simulink model "PR_Planar_Testbench_2018"  (R2024a)
settings: Solver=FixedStepDiscrete  StartTime=0.0  StopTime=inf  FixedStep=param.t_sample  RelTol=1e-3
undefined symbols (not defined in the file): max_qa, min_qa, param, slave3
libraries: Cust_Library_planarPKM x54, simulink_extras x27, dspswit3 x24, simulink x22, etherlab_lib x12
(part 5 of 6)

== system PR_Planar_Testbench_2018/Communication/Klemmen zu Simulink/int in double1 ==
  pos_raw : Inport
  current_raw : Inport  Port=2
  Constant : Constant  Value=param.t_sample  SampleTime=-1
  Delay1 : Delay  DelayLength=1  InitialCondition=param.offset_qa2_rad
  Delay4 : Delay  DelayLength=1
  MATLAB Function1 : MATLAB Function  TreatAsAtomicUnit=on
  Position_i1 : Gain  Gain=(2*pi)/(2^(20))  ParamDataTypeStr=float('double')  OutDataTypeStr=float('double')
  Sum1 : Sum  Inputs=|+-
  Torque_i1 : Gain  Gain=(6.6116*16.5)/3280  ParamDataTypeStr=float('double')  OutDataTypeStr=float('double')
  int16_2_double : DataTypeConversion  OutDataTypeStr=double  SaturateOnIntegerOverflow=off  RndMeth=Floor
  offset_s1 : Constant  Value=param.offset_qa2_rad  SampleTime=-1
  pos_Achse12 : DataTypeConversion  OutDataTypeStr=double  SaturateOnIntegerOverflow=off  RndMeth=Floor
  pos : Outport
  vel : Outport  Port=2
  acc : Outport  Port=3
  tau : Outport  Port=4
  wires:
  current_raw/1 -> int16_2_double/1
  Constant/1 -> MATLAB Function1/4(t_sample)
  Delay4/1 -> MATLAB Function1/3(prev_vel)
  pos_raw/1 -> pos_Achse12/1
  MATLAB Function1/1(vel) -> Delay4/1, vel/1  "dq"
  Delay1/1 -> MATLAB Function1/2(prev_pos)
  MATLAB Function1/2(acc) -> acc/1
  Torque_i1/1 -> tau/1  "tau_mess_RD1"
  pos_Achse12/1 -> Position_i1/1
  offset_s1/1 -> Sum1/2
  Position_i1/1 -> Sum1/1
  Sum1/1 -> pos/1, Delay1/1, MATLAB Function1/1(u)
  int16_2_double/1 -> Torque_i1/1

== system PR_Planar_Testbench_2018/Communication/Klemmen zu Simulink/int in double2 ==
  pos_raw : Inport
  current_raw : Inport  Port=2
  Constant : Constant  Value=param.t_sample  SampleTime=-1
  Delay1 : Delay  DelayLength=1  InitialCondition=param.offset_qa3_rad
  Delay4 : Delay  DelayLength=1
  MATLAB Function1 : MATLAB Function  TreatAsAtomicUnit=on
  Position_i1 : Gain  Gain=(2*pi)/(2^(20))  ParamDataTypeStr=float('double')  OutDataTypeStr=float('double')
  Sum1 : Sum  Inputs=|+-
  Torque_i1 : Gain  Gain=(6.7315*16.5)/3280  ParamDataTypeStr=float('double')  OutDataTypeStr=float('double')
  int16_2_double : DataTypeConversion  OutDataTypeStr=double  SaturateOnIntegerOverflow=off  RndMeth=Floor
  offset_s1 : Constant  Value=param.offset_qa3_rad  SampleTime=-1
  pos_Achse12 : DataTypeConversion  OutDataTypeStr=double  SaturateOnIntegerOverflow=off  RndMeth=Floor
  pos : Outport
  vel : Outport  Port=2
  acc : Outport  Port=3
  tau : Outport  Port=4
  wires:
  current_raw/1 -> int16_2_double/1
  Constant/1 -> MATLAB Function1/4(t_sample)
  Delay4/1 -> MATLAB Function1/3(prev_vel)
  pos_raw/1 -> pos_Achse12/1
  MATLAB Function1/1(vel) -> Delay4/1, vel/1  "dq"
  Delay1/1 -> MATLAB Function1/2(prev_pos)
  MATLAB Function1/2(acc) -> acc/1
  Torque_i1/1 -> tau/1  "tau_mess_RD1"
  pos_Achse12/1 -> Position_i1/1
  offset_s1/1 -> Sum1/2
  Position_i1/1 -> Sum1/1
  Sum1/1 -> pos/1, Delay1/1, MATLAB Function1/1(u)
  int16_2_double/1 -> Torque_i1/1

== system PR_Planar_Testbench_2018/Logic/Trajectory/Acceleration ==
  tr_run : Inport
  Counter : Inport  Port=2
  traj_length : Inport  Port=3
  Constant1 : Constant  Value=0  SampleTime=-1
  Less Than : RelationalOperator  Operator=<  OutDataTypeStr=boolean  RndMeth=Simplest  InputSameDT=off
  Mux : Mux  Inputs=3
  OR : Logic  AllPortsSameDT=off  OutDataTypeStr=boolean
  PhieDD : Constant  Value=0  SampleTime=-1
  Saturation : Saturate  UpperLimit=param.len_traj_init-1  LowerLimit=0
  Selector : Selector  IndexMode=Zero-based  IndexOptions=Index vector (port)  Indices=[1 3]  OutputSizes=1
  Selector1 : Selector  IndexMode=Zero-based  IndexOptions=Index vector (port)  Indices=[1 3]  OutputSizes=1
  Selector2 : Selector  IndexMode=Zero-based  IndexOptions=Index vector (port)  Indices=[1 3]  OutputSizes=1
  Switch : Switch  Criteria=u2 > Threshold  SaturateOnIntegerOverflow=off  InputSameDT=off
  XDD : Constant  Value=0  SampleTime=-1
  YDD : Constant  Value=0  SampleTime=-1
  XDDE_soll : Outport
  wires:
  Constant1/1 -> Switch/3
  traj_length/1 -> Less Than/2
  Selector2/1 -> Mux/3
  PhieDD/1 -> Selector2/1
  Selector1/1 -> Mux/2
  Counter/1 -> Switch/1, Less Than/1
  XDD/1 -> Selector/1
  Switch/1 -> Saturation/1
  Less Than/1 -> OR/2
  OR/1 -> Switch/2
  Selector/1 -> Mux/1
  YDD/1 -> Selector1/1
  Mux/1 -> XDDE_soll/1
  tr_run/1 -> OR/1
  Saturation/1 -> Selector2/2, Selector1/2, Selector/2

== system PR_Planar_Testbench_2018/Logic/Trajectory/Pose ==
  tr_run : Inport
  Counter : Inport  Port=2
  traj_length : Inport  Port=3
  AND : Logic  AllPortsSameDT=off  OutDataTypeStr=boolean
  AND1 : Logic  AllPortsSameDT=off  OutDataTypeStr=boolean
  Constant1 : Constant  Value=0  SampleTime=-1
  Constant5 : Constant  Value=0  SampleTime=-1
  Delay1 : Delay  DelayLength=1
  Equal : RelationalOperator  Operator=~=  OutDataTypeStr=boolean  RndMeth=Simplest  InputSameDT=off
  Less Than : RelationalOperator  Operator=<  OutDataTypeStr=boolean  RndMeth=Simplest  InputSameDT=off
  Mux : Mux  Inputs=3
  Mux1 : Mux  Inputs=3
  Phie : Constant  Value=0  SampleTime=-1
  Phie0 : Constant  Value=0  SampleTime=-1
  Saturation : Saturate  UpperLimit=param.len_traj_init-1  LowerLimit=0
  Scope : Scope  NumInputPorts=2
  Scope1 : Scope  NumInputPorts=3
  Scope2 : Scope  NumInputPorts=2
  Scope3 : Scope
  Selector{,1..3} (4 alike) : Selector  IndexMode=Zero-based  IndexOptions=Index vector (port)  Indices=[1 3]  OutputSizes=1
  Switch : Switch  Criteria=u2 > Threshold  SaturateOnIntegerOverflow=off  InputSameDT=off
  X : Constant  Value=0  SampleTime=-1
  X0 : Constant  Value=0  SampleTime=-1
  Y : Constant  Value=0  SampleTime=-1
  Y0 : Constant  Value=0  SampleTime=-1
  isValid : Constant  Value=0  SampleTime=-1
  XE_soll : Outport
  tr_isCalculating : Outport  Port=2
  XE0_soll : Outport  Port=3
  tr_valid : Outport  Port=4
  wires:
  Constant1/1 -> Switch/3
  traj_length/1 -> Less Than/2
  Selector2/1 -> Mux/3
  Phie/1 -> Selector2/1
  Selector1/1 -> Mux/2
  Counter/1 -> Scope1/1, Switch/1, Less Than/1, Scope3/1
  Selector/1 -> Mux/1
  Constant5/1 -> Equal/1
  Switch/1 -> Saturation/1, Equal/2
  Less Than/1 -> Scope1/3, AND/2
  AND/1 -> Switch/2
  Mux/1 -> XE_soll/1
  Mux1/1 -> XE0_soll/1
  Equal/1 -> Scope2/2, AND1/2
  Y/1 -> Selector1/1
  tr_run/1 -> Scope1/2, AND/1, Scope2/1, AND1/1
  Y0/1 -> Mux1/2
  X0/1 -> Mux1/1
  Phie0/1 -> Mux1/3
  Saturation/1 -> Scope/2, Selector3/2, Selector/2, Selector1/2, Selector2/2
  AND1/1 -> tr_isCalculating/1, Scope/1
  X/1 -> Selector/1
  isValid/1 -> Selector3/1
  Selector3/1 -> Delay1/1
  Delay1/1 -> tr_valid/1

== system PR_Planar_Testbench_2018/Logic/Trajectory/Velocity ==
  tr_run : Inport
  Counter : Inport  Port=2
  traj_length : Inport  Port=3
  Constant1 : Constant  Value=0  SampleTime=-1
  Display : Display
  Less Than : RelationalOperator  Operator=<  OutDataTypeStr=boolean  RndMeth=Simplest  InputSameDT=off
  Mux : Mux  Inputs=3
  OR : Logic  AllPortsSameDT=off  OutDataTypeStr=boolean
  PhieD : Constant  Value=0  SampleTime=-1
  Saturation : Saturate  UpperLimit=param.len_traj_init-1  LowerLimit=0
  Scope : Scope
  Selector : Selector  IndexMode=Zero-based  IndexOptions=Index vector (port)  Indices=[1 3]  OutputSizes=1
  Selector1 : Selector  IndexMode=Zero-based  IndexOptions=Index vector (port)  Indices=[1 3]  OutputSizes=1
  Selector2 : Selector  IndexMode=Zero-based  IndexOptions=Index vector (port)  Indices=[1 3]  OutputSizes=1
  Switch : Switch  Criteria=u2 > Threshold  SaturateOnIntegerOverflow=off  InputSameDT=off
  XD : Constant  Value=0  SampleTime=-1
  YD : Constant  Value=0  SampleTime=-1
  XDE_soll : Outport
  wires:
  Mux/1 -> XDE_soll/1
  YD/1 -> Selector1/1
  Selector/1 -> Mux/1
  OR/1 -> Switch/2
  Less Than/1 -> OR/2
  tr_run/1 -> OR/1
  Switch/1 -> Saturation/1
  XD/1 -> Selector/1
  Counter/1 -> Switch/1, Less Than/1
  Selector1/1 -> Mux/2
  PhieD/1 -> Selector2/1
  Selector2/1 -> Mux/3
  traj_length/1 -> Less Than/2
  Constant1/1 -> Switch/3
  Saturation/1 -> Display/1, Scope/1, Selector/2, Selector1/2, Selector2/2

== system PR_Planar_Testbench_2018/Logic/Validation of the EE end target pose/valid_invers_kinematic1 ==
  theta_in : Inport
  AND_Theta1 : Logic  Commented=on  AllPortsSameDT=off  OutDataTypeStr=boolean
  AND_Theta2 : Logic  Commented=on  AllPortsSameDT=off  OutDataTypeStr=boolean
  AND_Theta3 : Logic  Commented=on  AllPortsSameDT=off  OutDataTypeStr=boolean
  AND_Theta4 : Logic  Commented=on  Inputs=3  AllPortsSameDT=off  OutDataTypeStr=boolean
  Constant : Constant  Value=param.min_qa  SampleTime=-1
  Constant1 : Constant  Value=param.max_qa  SampleTime=-1
  Demux : Demux  Commented=on  Outputs=3
  MATLAB Function : MATLAB Function  TreatAsAtomicUnit=on
  Radians to Degrees : simulink_extras/Transformations/Radians to Degrees
  max_theta1 : simulink/Logic and Bit Operations/Compare To Constant  Commented=on  relop=<=  const=max_qa(1)  OutDataTypeStr=boolean
  max_theta4 : simulink/Logic and Bit Operations/Compare To Constant  Commented=on  relop=<=  const=max_qa(2)  OutDataTypeStr=boolean
  max_theta5 : simulink/Logic and Bit Operations/Compare To Constant  Commented=on  relop=<=  const=max_qa(3)  OutDataTypeStr=boolean
  min_theta1 : simulink/Logic and Bit Operations/Compare To Constant  Commented=on  relop=>=  const=min_qa(1)  OutDataTypeStr=boolean
  min_theta4 : simulink/Logic and Bit Operations/Compare To Constant  Commented=on  relop=>=  const=min_qa(2)  OutDataTypeStr=boolean
  min_theta5 : simulink/Logic and Bit Operations/Compare To Constant  Commented=on  relop=>=  const=min_qa(3)  OutDataTypeStr=boolean
  kinematic_valid : Outport  VectorParamsAs1DForOutWhenUnconnected=off
  wires:
  AND_Theta3/1 -> AND_Theta4/3
  AND_Theta2/1 -> AND_Theta4/2
  AND_Theta1/1 -> AND_Theta4/1
  Demux/2 -> max_theta4/1, min_theta4/1
  Demux/3 -> max_theta5/1, min_theta5/1
  Demux/1 -> min_theta1/1, max_theta1/1
  max_theta4/1 -> AND_Theta2/2
  min_theta4/1 -> AND_Theta2/1
  min_theta1/1 -> AND_Theta1/1
  max_theta5/1 -> AND_Theta3/2
  min_theta5/1 -> AND_Theta3/1
  max_theta1/1 -> AND_Theta1/2
  Radians to Degrees/1 -> MATLAB Function/1(u), Demux/1
  theta_in/1 -> Radians to Degrees/1
  MATLAB Function/1(y) -> kinematic_valid/1
  Constant/1 -> MATLAB Function/2(min_qa)
  Constant1/1 -> MATLAB Function/3(max_qa)

== matlab function PR_Planar_Testbench_2018/Logic/MATLAB Function11 ==
  data: Init_Reaction input; x_des_retr_m_rad output; n_f input; x input; d_retr_m input; phi_retr_deg input; sign_grad_qp_phiz input
function x_des_retr_m_rad = fcn(Init_Reaction, n_f, x, d_retr_m, phi_retr_deg, sign_grad_qp_phiz)
    if Init_Reaction
        delta_x = [n_f(1)*d_retr_m; n_f(2)*d_retr_m; -deg2rad(phi_retr_deg)*sign_grad_qp_phiz(1)];
        x_des_retr_m_rad = x + delta_x;
    else
        x_des_retr_m_rad = x; 
    end
end

== matlab function PR_Planar_Testbench_2018/Logic/MATLAB Function12 ==
  data: Init_Reac input; Init_Retr_valid output; x_soll_retr_m_rad input; param parameter
function Init_Retr_valid = fcn(Init_Reac, x_soll_retr_m_rad, param)

r = sqrt(x_soll_retr_m_rad(1)^2+x_soll_retr_m_rad(2)^2);

if Init_Reac && r <= param.max_radius && abs(x_soll_retr_m_rad(3))< param.max_phie
    Init_Retr_valid = true; 
else 
    Init_Retr_valid = false;
end

== matlab function PR_Planar_Testbench_2018/Controlpanel/MATLAB Function ==
  data: Statusword_S1 input; Statusword output; Statusword_S2 input; Statusword_S3 input; Statusword_Trans_Drive input
function Statusword  = fcn(Statusword_S1, Statusword_S2, Statusword_S3, Statusword_Trans_Drive)
if Statusword_S1 == Statusword_S2 && Statusword_S1 == Statusword_S3 && Statusword_S1 == Statusword_Trans_Drive
    Statusword = Statusword_S1;
else
    Statusword = 0;
end

== matlab function PR_Planar_Testbench_2018/Init_Block/MATLAB Function ==
  data: Controlword_S1 input; Controlword output; Controlword_S2 input; Controlword_S3 input
function Controlword  = fcn(Controlword_S1, Controlword_S2, Controlword_S3)
if Controlword_S1 == Controlword_S2 && Controlword_S1 == Controlword_S3
    Controlword = Controlword_S1;
else
    Controlword = uint16(0);
end

== matlab function PR_Planar_Testbench_2018/Logic/MATLAB Function13 ==
  data: state input; y output; x_des_bp input; x_des_retr input; retraction_active output
function [y, retraction_active] = fcn(state, x_des_bp, x_des_retr)
if state == 26 || state == 27
    y = x_des_retr;
    retraction_active = 1;
else % state == 3 || state == 4 || state == 8 || state == 9
    y = x_des_bp;
    retraction_active = 0;
end

== matlab function PR_Planar_Testbench_2018/Communication/Klemmen zu Simulink/Uint in double/MATLAB Function1 ==
  data: u input; vel output; prev_pos input; prev_vel input; t_sample input; acc output
function [vel, acc] = fcn(u, prev_pos, prev_vel, t_sample)

vel = (u-prev_pos)/t_sample;
acc = (vel-prev_vel)/t_sample;

== matlab function PR_Planar_Testbench_2018/Communication/Klemmen zu Simulink/Uint in double/MATLAB Function2 ==
  data: u_uint input; y output
function y = fcn(u_uint)
% für uint16 folgt: 
 
tmp = 2^16; % = 65536  
% error = (setPoint + 512 - currPos) % 1024 - 512;
% // Calculation
% error = (1023 + 512 - 10) % 1024 - 512
%       = 1525 % 1024 - 512
%       = 501 - 512
%       = -11
% u=uint16(10)
% u2 = double(u)
% c = 2+u
% prev = 0;
% y = mod( ( (tmp-1) + tmp/2 - u), tmp) - tmp/2
% y = mod(u, tmp) - tmp/2
u = double(u_uint);
y =  (mod( ( tmp/2 + u), tmp) - (tmp)/2);
% 
% if (u-prev)>=0 % kein Über- oder Unterlauf
%    y = u; 
% elseif (u-prev)<0 % Über- oder Unterlauf
%    
%     if prev == 0 % Unterlauf
%         y = 
%     elseif prev == tmp-1 % Überlauf
%     
%     end
% end

% tmp2 = [];
% 
% for u_tmp = 0:1:2^16-1
%    tmp2 = [tmp2; mod( ( tmp/2 + u_tmp), tmp) - (tmp)/2]; 
% end
% plot(tmp2);

== matlab function PR_Planar_Testbench_2018/Communication/Klemmen zu Simulink/int in double/MATLAB Function1 ==
  data: u input; vel output; prev_pos input; prev_vel input; t_sample input; acc output
function [vel, acc] = fcn(u, prev_pos, prev_vel, t_sample)

vel = (u-prev_pos)/t_sample;
acc = (vel-prev_vel)/t_sample;

== matlab function PR_Planar_Testbench_2018/Communication/Klemmen zu Simulink/int in double1/MATLAB Function1 ==
  data: u input; vel output; prev_pos input; prev_vel input; t_sample input; acc output
function [vel, acc] = fcn(u, prev_pos, prev_vel, t_sample)

vel = (u-prev_pos)/t_sample;
acc = (vel-prev_vel)/t_sample;

== matlab function PR_Planar_Testbench_2018/Communication/Klemmen zu Simulink/int in double2/MATLAB Function1 ==
  data: u input; vel output; prev_pos input; prev_vel input; t_sample input; acc output
function [vel, acc] = fcn(u, prev_pos, prev_vel, t_sample)

vel = (u-prev_pos)/t_sample;
acc = (vel-prev_vel)/t_sample;

== matlab function PR_Planar_Testbench_2018/Control/MATLAB Function4 ==
  data: u input; y output
function y = fcn(u)

y = diag(u);

== matlab function PR_Planar_Testbench_2018/Communication/MATLAB Function ==
  data: Statusword_S1 input; Statusword output; Statusword_S2 input; Statusword_S3 input; Statusword_TranslDrive input
function Statusword  = fcn(Statusword_S1, Statusword_S2, Statusword_S3, Statusword_TranslDrive)
if Statusword_S1 == Statusword_S2 && Statusword_S1 == Statusword_S3 && Statusword_S1 == Statusword_TranslDrive
    Statusword = Statusword_S1;
else
    Statusword = uint16(0);
end

== matlab function PR_Planar_Testbench_2018/Logic/Validation of the EE end target pose/kinematic_invers ==
  data: xEE input; qa output; qp output; param parameter
function [qa, qp] = calcq_(xEE, param)
[qa, qp] = calcq(xEE, param.psi_j, param.beta_j, param.r_fixPlat_j, param.r_mobPlat_j, param.l_all_id);
end

== matlab function PR_Planar_Testbench_2018/DirectDynamics_MuJoCo/Planare PKM mit Kapsel ==
  data: capspos input; tau input; q output; qd output; qdd output; param parameter
function [q, qd, qdd] = call_mujoco(capspos, tau, param)
    % Funktion für den Mujoco-Aufruf und -Ausgabe der kinematischen Größen
    % Eingabe:
    % capspos in m und m/s: Kapsenposition und -geschwindigkeit [posx velx posy vely] (4x1)
    % tau in Nm: Antriebsmomente in Antriebskoordinaten (3x1)
    %
    % Ausgabe:
    % q_ in m und rad: Vektor der Kapsel-, Gelenk- und Plattformkoordinaten (14x1)
    % qd_ in m/s und rad/s: Vektor der Kapsel-, Gelenk- und Plattformgeschwindigkeiten (14x1)
    % qdd_ in m/s^2 und rad/s^2: Vektor der Kapsel-, Gelenk- und Plattformbeschleunigungen (14x1)
    
    % Aran Mohammad, aran.mohammad@imes.uni-hannover.de, 2022-12
    % (C) Institut für Mechatronische Systeme, Universität Hannover
    
%#codegen
coder.extrinsic('mjx');
coder.extrinsic('evalin');
mjx('set', 'ctrl', [capspos' tau']);

mjx('step', param.t_sample/0.001);

q_ = zeros(14,1); 
qd = zeros(14,1); 
qdd = zeros(14,1);

qoffset =[0.4; 0.3;
     25.5184; 122.3049; -237.8233; ...
     0; 0; 0; ...
     25.9632; 121.7747; -358.5010; ...
     24.3787; 124.6086; -479.4775]*pi/180;

q_ = mjx('get', 'qpos');
q = q_ + qoffset;
qd = mjx('get', 'qvel');
qdd = mjx('get', 'qacc');

== matlab function PR_Planar_Testbench_2018/DirectDynamics_MuJoCo/Contact_data_Mujoco2Simulink ==
  data: n output; pos output size=[4 3]; frame output size=[4 9]; dist output size=[4 1]; force output size=[4 6]; geom1 output size=[4 1]; geom2 output size=[4 1]
function [n, pos, frame, dist, force, geom1, geom2]  = call_mujoco()
    % Funktion für den Aufrung der Mujoco-Größen
    %
    % Ausgabe:
    % n: Anzahl der Kontaktpunkte (1x1)
    % pos in m: Globale Koordinaten der Kontaktpunkte (nx1)
    % fram: Kontaktframe in globalen Koordinaten (row-major Format, 1. Achse ist die Kraftnormale) (nx9)
    % dist: Abstand der involvierten Oberflaechen, negativ bedeutet Durchdringung (nx1)
    % force: Kraft im Kontaktframe (nx6)
    % geom1: Index der ersten Kontaktgeometrie (nx1)
    % geom2: Index der zweiten Kontaktgeometrie, die Kraft zeigt von Geometrie 1 zu Geometrie 2 (nx1)
    
    % Aran Mohammad, aran.mohammad@imes.uni-hannover.de, 2022-12
    % (C) Institut für Mechatronische Systeme, Universität Hannover

%#codegen
coder.extrinsic('mj_read_contacts_test');
n=0;
pos = zeros(n,3);
frame = zeros(n,9);
dist = zeros(n,1);
force = zeros(n,6);
geom1 = zeros(n,1);
geom2 = zeros(n,1);

[n, pos, frame, dist, force, geom1, geom2] = mj_read_contacts_test();

== matlab function PR_Planar_Testbench_2018/Logic/MATLAB Function1 ==
  data: EE_act input; TR_in_starting_pos output; vec_traj_0 input
function TR_in_starting_pos = fcn(EE_act, vec_traj_0)
%#codegen


    tol_starting_pose = 0.004;
    
    if abs(EE_act(1) - vec_traj_0(1)) < tol_starting_pose && abs(EE_act(2) - vec_traj_0(2)) < tol_starting_pose && abs(EE_act(3) - vec_traj_0(3)) < 2.5*tol_starting_pose
        TR_in_starting_pos = 1;
    else
        TR_in_starting_pos = 0;
    end
% y=0;
end

== matlab function PR_Planar_Testbench_2018/Communication/Klemmen zu Simulink/MATLAB Function4 ==
  data: u input; vel output; prev_pos input; prev_vel input; t_sample input; acc output
function [vel, acc] = fcn(u, prev_pos, prev_vel, t_sample)

vel = (u-prev_pos)/t_sample;
acc = (vel-prev_vel)/t_sample;

== matlab function PR_Planar_Testbench_2018/Kinematics/MATLAB Function6 ==
  data: q input; y output; x input; qp2D_correct input
function y = fcn(q, x, qp2D_correct)
% Achtung: ohne psi_j, da auf Geschwindigkeit- und Beschleunigungsebene
% (und psi_j=const--> d_psi_j=0)
y_=zeros(9,1);
q13 = x(3) - (q(1,1) + q(2,1)); 
q23 = x(3) - (q(3,1) + qp2D_correct); 
q33 = x(3) - (q(5,1) + q(6,1)); 

y_ = [q(1,1); q(2,1); q13; ...
     q(3,1); qp2D_correct; q23; ...
     q(5,1); q(6,1); q33];
y=y_;

== matlab function PR_Planar_Testbench_2018/Logic/Safety functions/MATLAB Function ==
  data: u1 input; y output; u2 input; u3 input; u4 input; u5 input; u6 input; u7 input; u8 input; u9 input; u10 input; u11 input
function y = fcn(u1, u2, u3, u4, u5, u6, u7, u8, u9, u10, u11)
    % Find out which error is present
    % A 1 at index i in y indicates that the i-th error occurs
    
    y_tmp = ones(11,1); % Initialization with all active errors. Redundant 
    
    if u1 == 0 
        y_tmp(1,1) = 0;
    end
    
    if u2 == 0
        y_tmp(2,1) = 0;
    end
    
    if u3 == 0
        y_tmp(3,1) = 0;
    end
    
    if u4 == 0
        y_tmp(4,1) = 0;
    end
    
    if u5 == 0
        y_tmp(5,1) = 0;
    end
    if u6 == 0
        y_tmp(6,1) = 0;
    end
    if u7 == 0
        y_tmp(7,1) = 0;
    end
    if u8 == 0
        y_tmp(8,1) = 0;
    end
    if u9 == 0
        y_tmp(9,1) = 0;
    end
    if u10 == 0
        y_tmp(10,1) = 0;
    end
    if u11 == 0
        y_tmp(11,1) = 0;
    end
    y = y_tmp;

== matlab function PR_Planar_Testbench_2018/Control/MATLAB Function5 ==
  data: u input; y output
function y = fcn(u)

y = diag(u);

== matlab function PR_Planar_Testbench_2018/Control/MATLAB Function6 ==
  data: u input; y output
function y = fcn(u)

y = diag(u);

== matlab function PR_Planar_Testbench_2018/Observer/MATLAB Function3 ==
  data: u input; norm_u output
function norm_u = fcn(u)

norm_u = norm(u);

== matlab function PR_Planar_Testbench_2018/Communication/Klemmen zu Simulink/MATLAB Function5 ==
  data: u input; vel output; prev_pos input; prev_vel input; t_sample input; acc output
function [vel, acc] = fcn(u, prev_pos, prev_vel, t_sample)

vel = (u-prev_pos)/t_sample;
acc = (vel-prev_vel)/t_sample;

== matlab function PR_Planar_Testbench_2018/Kinematics/MATLAB Function2 ==
  data: u input; y output
function y = xEE_3dTo6D(u)

y = [u(1); u(2); 0;0;0; u(3)];

== matlab function PR_Planar_Testbench_2018/Kinematics/MATLAB Function3 ==
  data: u input; y output
function y = xEE_3dTo6D(u)

y = [u(1); u(2); 0;0;0; u(3)];

== matlab function PR_Planar_Testbench_2018/Kinematics/MATLAB Function4 ==
  data: u input; y output
function y = xEE_3dTo6D(u)

y = [u(1); u(2); 0;0;0; u(3)];

== matlab function PR_Planar_Testbench_2018/Logic/MATLAB Function22 ==
  data: Init_reaction input; clamping_det input; qap_retr_soll output; clampBody input; qa input; q input; d_retr_cl1 input; d_retr_cl2 input; J_qap output; Jinv_hq_qa input; qap_retr output; tauext_obs input
function [qap_retr_soll, J_qap, qap_retr] = fcn(Init_reaction, clamping_det, clampBody, qa, q, d_retr_cl1, d_retr_cl2, Jinv_hq_qa, tauext_obs)
    
    qp_contact = q([2 5 8]);
    
    if Init_reaction && clamping_det
        qap_retr = [qa(clampBody); qp_contact(clampBody)];
        qa_retr = qa(clampBody) + sign(tauext_obs(clampBody))*d_retr_cl1/0.5;
        J_xpqa_link1 = zeros(1,3);
        J_xpqa_link1(1,clampBody) = 1;
        qp_retr = qp_contact(clampBody) - d_retr_cl2/0.5;
        Jinv_qp_qa = Jinv_hq_qa(2+3*(clampBody-1),:);
    else
        qa_retr = qa(1);
        qp_retr = qp_contact(1);
        J_xpqa_link1 = zeros(1,3);
        Jinv_qp_qa = zeros(1,3);
        qap_retr = [qa(1); qp_contact(1)];
    end

    qap_retr_soll = [qa_retr; qp_retr];
    J_qap = [J_xpqa_link1; Jinv_qp_qa];

== matlab function PR_Planar_Testbench_2018/Logic/MATLAB Function ==
  data: u input; y output
function y = xEE_3dTo6D(u)

y = [u(1); u(2); 0;0;0; u(3)];

== matlab function PR_Planar_Testbench_2018/Logic/MATLAB Function2 ==
  data: u input; y output
function y = xEE_3dTo6D(u)

y = [u(1); u(2); 0;0;0; u(3)];

== matlab function PR_Planar_Testbench_2018/Logic/MATLAB Function3 ==
  data: u input; y output
function y = xEE_3dTo6D(u)

y = [u(1); u(2); 0;0;0; u(3)];

== matlab function PR_Planar_Testbench_2018/Communication/Klemmen zu Simulink/MATLAB Function6 ==
  data: u input; vel output; prev_pos input; prev_vel input; t_sample input; acc output
function [vel, acc] = fcn(u, prev_pos, prev_vel, t_sample)

vel = (u-prev_pos)/t_sample;
acc = (vel-prev_vel)/t_sample;

== matlab function PR_Planar_Testbench_2018/Communication/MATLAB Function3 ==
  data: u input; y output; u2 input
function y = fcn(u, u2)
if u2 == 1
    if u == 37896
       y = 128;
    else
       y=0;
    end
else
    y=0;
end

== matlab function PR_Planar_Testbench_2018/Kinematics/MATLAB Function ==
  data: q input; y output; x input
function y = fcn(q, x)
% Achtung: ohne psi_j, da auf Geschwindigkeit- und Beschleunigungsebene
% (und psi_j=const--> d_psi_j=0)
q13 = x(3) - (q(1,1) + q(2,1)); 
q23 = x(3) - (q(3,1) + q(4,1)); 
q33 = x(3) - (q(5,1) + q(6,1)); 

y = [q(1,1); q(2,1); q13; ...
     q(3,1); q(4,1); q23; ...
     q(5,1); q(6,1); q33];

== matlab function PR_Planar_Testbench_2018/Kinematics/MATLAB Function1 ==
  data: q input; y_final output; x input; qp2DD_correct input
function y_final = fcn(q, x, qp2DD_correct)
% Achtung: ohne psi_j, da auf Geschwindigkeit- und Beschleunigungsebene
% (und psi_j=const--> d_psi_j=0)
% q13 = x(3) - (q(1,1) + q(2,1)); 
% q23 = x(3) - (q(3,1) + qp2DD_correct); 
% q33 = x(3) - (q(5,1) + q(6,1)); 
% 
% y = [q(1,1); q(2,1); q13; ...
%      q(3,1); qp2DD_correct; q23; ...
%      q(5,1); q(6,1); q33];
 % Achtung: ohne psi_j, da auf Geschwindigkeit- und Beschleunigungsebene
% (und psi_j=const--> d_psi_j=0)
y_=zeros(9,1);
q13 = x(3) - (q(1,1) + q(2,1)); 
q23 = x(3) - (q(3,1) + qp2DD_correct); 
q33 = x(3) - (q(5,1) + q(6,1)); 

y_ = [q(1,1); q(2,1); q13; ...
     q(3,1); qp2DD_correct; q23; ...
     q(5,1); q(6,1); q33];
 y_final=y_;

== matlab function PR_Planar_Testbench_2018/Control/MATLAB Function7 ==
  data: tau_ir input; tau_rr input; rr_level input; data input; tau_out output size=[3,1]; tau_prev input; param parameter
function tau_out = fcn(tau_ir, tau_rr, rr_level, data, tau_prev, param)

    if rr_level == 1 || rr_level == 2 || rr_level == 3 
        tau_out = tau_rr;%lim_in(tau, tau_prev, param.delta_tau_max_Nm);
    elseif rr_level == 0
        tau_out = tau_ir;
    else
        tau_out = zeros(3,1);
    end
end

== matlab function PR_Planar_Testbench_2018/Control/MATLAB Function ==
  data: u input; y output; not_defined_nan input
function y = fcn(u, not_defined_nan)

if isnan(sum(u)) || not_defined_nan > 0 || isinf(sum(u)) || sum(isinf(u))>0 || sum(isnan(u))>0
    y = [0;0;0];
else
    y=u;
end

== matlab function PR_Planar_Testbench_2018/Control/MATLAB Function1 ==
  data: u input; y output
function y = fcn(u)

if isnan(sum(u))
    y = [0;0;0];
else
    y=u;
end

== matlab function PR_Planar_Testbench_2018/Logic/MATLAB Function7 ==
  data: control_out input; turn_control_off output
function turn_control_off = fcn(control_out)
% Wenn Ist-Werte als Soll-Werte vorgegeben werden, dann soll der Regler
% einen Ausgang=0 haben. Das ist für den Stillstand gedacht

if control_out==0
    turn_control_off=1;
else
    turn_control_off=0;
end

== matlab function PR_Planar_Testbench_2018/Logic/MATLAB Function4 ==
  data: u input; y output
function y = fcn(u)
if u == 3 || u == 4 || u == 8 || u == 9 || u == 26 || u == 27
    y = 0;
else
    y = 1;
end

== matlab function PR_Planar_Testbench_2018/Control/MATLAB Function2 ==
  data: torque_desired input; y output; turn_control_off input
 function y = fcn(torque_desired, turn_control_off)
if turn_control_off==1
    y=[0;0;0];
else
    y=torque_desired;
end

== matlab function PR_Planar_Testbench_2018/DirectDynamics_MuJoCo/MATLAB Function4 ==
  data: Fext_link_KSGj output; q input; predBody input; Fext_links_KS0 input size=[6 1]; param parameter
function Fext_link_KSGj = fcn(q, predBody, Fext_links_KS0, param)
    Fext_link_KSGj=zeros(3,1);
    Fext_link_KS0 = Fext_links_KS0(1:3);
    if predBody == 2 
        pred_chain = 1; 
    elseif predBody == 4 
        pred_chain = 2; 
    elseif predBody == 6 
        pred_chain = 3; 
    else
        Fext_link_KSGj=zeros(3,1);
        return
    end
    qa = q([1 4 7]);
    qp = q([2 5 8]);
    qseg = qa(pred_chain) + param.psi_j(pred_chain)+qp(pred_chain);    
    R_0Gj = [cos(qseg) -sin(qseg) 0 ; sin(qseg) cos(qseg) 0 ;0 0 1]; 
    Fext_link_KSGj = R_0Gj' * Fext_link_KS0;

== matlab function PR_Planar_Testbench_2018/Control/TP1_impl/MATLAB Function16 ==
  data: u_raw input; u_filt output; u_prev input; a input; y_prev input; not_defined_nan output
function  [u_filt, not_defined_nan] = TP1_DiffEq(u_raw, u_prev, a, y_prev)
if isnan(sum(u_raw))
    u_filt = [0;0;0];
    not_defined_nan = 1;
elseif isnan(sum(TP1_DiffEq(u_raw, u_prev, a, y_prev)))
        u_filt = [0;0;0];
        not_defined_nan = 2;
else
    u_filt = TP1_DiffEq(u_raw, u_prev, a, y_prev);
    not_defined_nan = 0;
end

== matlab function PR_Planar_Testbench_2018/Logic/Validation of the EE end target pose/valid_invers_kinematic1/MATLAB Function ==
  data: u input; y output; min_qa input; max_qa input
function y = fcn(u, min_qa, max_qa)

if u(1)>=min_qa(1) && u(1)<=max_qa(1) && u(2)>=min_qa(2) && u(2)<=max_qa(2) && u(3)>=min_qa(3) && u(3)<=max_qa(3) 
    y=1;
else
    y=0;
end

== matlab function PR_Planar_Testbench_2018/Visualization/MATLAB Function ==
  data: u input; y output
function y = fcn(u)

y = diag(u);

== matlab function PR_Planar_Testbench_2018/Logic/isStandstill ==
  data: u input; y output
function y = fcn(u)
if u == 3 || u == 4 || u == 8 || u == 9 || u == 10 || u == 11 || u == 13 || u == 14
    y = 0;
else
    y = 1;
end

== matlab function PR_Planar_Testbench_2018/DirectDynamics_MuJoCo/MATLAB Function3 ==
  data: pos_contact_KSGj_2D output; nr_link input; s1 output; Fext_link1 output; Fext_link2 output; nr_chain input; q_rad input; pos_contacts_KS0_input input size=[4,3]; n input; s2 output; param parameter; frame_input input size=[4,9]; force_input input size=[4,6]; geom2 input size=[4,1]
function [pos_contact_KSGj_2D, s1, Fext_link1, Fext_link2, s2] = fcn(nr_link, nr_chain, q_rad, pos_contacts_KS0_input, n, param, ...
    frame_input, force_input, geom2)
    % Funktion für die Berechnung der längennormierten Kontaktorte und Linkkräfte in KS_0
    % Eingabe:
    % nr_link: Betroffenes Segment, 1 oder 2 (1x1)
    % nr_chain: Betroffene Beinkette, 1,2 oder 3 (1x1)
    % q_rad in rad: Vektor der Gelenkkoordinaten (9x1)
    % pos_contacts_KS0_input in m: Globale Koordinaten der Kontaktpunkte (nx1)
    % n: Anzahl der Kontaktpunkte (1x1)
    % frame_input: Kontaktframe in globalen Koordinaten (row-major Format, 1. Achse ist die Kraftnormale) (nx9)
    % force_input: Kraft im Kontaktframe (nx6)
    % geom2: Index der zweiten Kontaktgeometrie, die Kraft zeigt von Geometrie 1 zu Geometrie 2 (nx1)
    %
    % Ausgabe:
    % s1: Längennormierter Ort des ersten Kontaktortes im körperfesten KS (1x1)
    % Fext_link1: Kontaktkräfte am ersten Kontaktort in KS0 (3x1)
    % Fext_link2: Kontaktkräfte am ersten Kontaktort in KS0 (3x1)
    % s2: Längennormierter Ort des zweiten Kontaktortes im körperfesten KS(1x1)
    
    % Aran Mohammad, aran.mohammad@imes.uni-hannover.de, 2022-12
    % (C) Institut für Mechatronische Systeme, Universität Hannover
    
s1 = 0; % Normierter Angriffspunkt des ersten Kontaktes am Link
s2 = 0; % Normierter Angriffspunkt des zweiten Kontaktes am Link
Fext_link1 = zeros(3,1);
Fext_link2 = zeros(3,1);
pos_contact_KSGj_2D = zeros(2,1);
if n==1 && ismember( 17, geom2)
    frame_contact1 = [frame_input(1) frame_input(2) frame_input(3); 
                 frame_input(4) frame_input(5) frame_input(6); 
                 frame_input(7) frame_input(8) frame_input(9)]';
    Fext_link_KSContactframe = [force_input(1); force_input(2); force_input(3)];
    Fext_link1 = frame_contact1 * Fext_link_KSContactframe;
    Fext_link1(3)=0;
end
if n==1 && ~ismember( 17, geom2)
    pos_contact_KS0 = pos_contacts_KS0_input';
    pos_contact_KS0_2D = [pos_contact_KS0(1); pos_contact_KS0(2)];
    frame_contact1 = [frame_input(1) frame_input(2) frame_input(3); 
                 frame_input(4) frame_input(5) frame_input(6); 
                 frame_input(7) frame_input(8) frame_input(9)]';
    Fext_link_KSContactframe = [force_input(1); force_input(2); force_input(3)];
    qa = q_rad([1,4,7]);   
    qp = q_rad([2,5,8]);   

    % Direkte Kinematik der betrofffenen seriellen Kette mit Vektor von KS0 zu KS_Gj/KS_Fj
    posKS0_KS0_KSGj = [sin(param.psi_j(nr_chain));                -cos(param.psi_j(nr_chain))]*param.r_fixPlat_j(nr_chain);% Inertial zu Basisgelenk 1
    posKS0_KSGj_KS_Fj=[cos(param.psi_j(nr_chain) + qa(nr_chain));         sin(param.psi_j(nr_chain) + qa(nr_chain))]*param.l_all_id(nr_chain*2-1);% Basisgelenk1 zu Elle 1

    if nr_link == 1      
        q = qa(nr_chain) + param.psi_j(nr_chain);
        posKS0_contact1_KS0_KSGj = pos_contact_KS0_2D - posKS0_KS0_KSGj;
    else
        posKS0_contact1_KS0_KSGj = pos_contact_KS0_2D - (posKS0_KS0_KSGj + posKS0_KSGj_KS_Fj);
        q = qa(nr_chain) + param.psi_j(nr_chain)+qp(nr_chain);        
    end      
    
    R_0Gj = [cos(q) -sin(q) 0 ; sin(q) cos(q) 0 ;0 0 1];     
    pos_contact_KSGj_2D = R_0Gj(1:2,1:2)' * pos_contact_KS0_2D;
    posKSGj_contact1_KS0_KSGj = R_0Gj(1:2,1:2)' * posKS0_contact1_KS0_KSGj;
    s1 = posKSGj_contact1_KS0_KSGj(1)/param.l_all(nr_link);
    Fext_link1 = frame_contact1 * Fext_link_KSContactframe;
    Fext_link1(3)=0;

elseif n==2
    pos_contact_KS0 = pos_contacts_KS0_input';
    pos_contact1_KS0_2D = [pos_contact_KS0(1,1); pos_contact_KS0(2,1)];
    pos_contact2_KS0_2D = [pos_contact_KS0(1,2); pos_contact_KS0(2,2)];

    frame_contact1 = [frame_input(1,1) frame_input(1,2) frame_input(1,3); 
                     frame_input(1,4) frame_input(1,5) frame_input(1,6); 
                     frame_input(1,7) frame_input(1,8) frame_input(1,9)]';    
    frame_contact2 = [frame_input(2,1) frame_input(2,2) frame_input(2,3); 
                 frame_input(2,4) frame_input(2,5) frame_input(2,6); 
                 frame_input(2,7) frame_input(2,8) frame_input(2,9)]';    

    Fext_link1_KSContactframe = [force_input(1,1); force_input(1,2); force_input(1,3)];
    Fext_link2_KSContactframe = [force_input(2,1); force_input(2,2); force_input(2,3)];
    
    qa = q_rad([1,4,7]);   
    qp = q_rad([2,5,8]);   
    
    % Direkte Kinematik der betrofffenen seriellen Kette mit Vektor von KS0 zu KS_Gj/KS_Fj
    posKS0_KS0_KSGj = [sin(param.psi_j(nr_chain));                -cos(param.psi_j(nr_chain))]*param.r_fixPlat_j(nr_chain);% Inertial zu Basisgelenk 1
    posKS0_KSGj_KS_Fj=[cos(param.psi_j(nr_chain) + qa(nr_chain));         sin(param.psi_j(nr_chain) + qa(nr_chain))]*param.l_all_id(nr_chain*2-1);% Basisgelenk1 zu Elle 1
    
    q1 = qa(nr_chain) + param.psi_j(nr_chain);
    R_0Gj_contact1 = [cos(q1) -sin(q1) 0 ; sin(q1) cos(q1) 0 ;0 0 1];     
    posKS0_contact1_KS0_KSGj = pos_contact1_KS0_2D - posKS0_KS0_KSGj;
    posKSGj_contact1_KS0_KSGj = R_0Gj_contact1(1:2,1:2)' * posKS0_contact1_KS0_KSGj;
    s1 = posKSGj_contact1_KS0_KSGj(1)/param.l_all(1);
    Fext_link1 = frame_contact1 * Fext_link1_KSContactframe;
    Fext_link1(3)=0;
    
    % Zweiter Kontakt
    q2 = qa(nr_chain) + param.psi_j(nr_chain)+qp(nr_chain);        
    R_0Gj_contact2 = [cos(q2) -sin(q2) 0 ; sin(q2) cos(q2) 0 ;0 0 1];     
    posKS0_contact2_KS0_KSGj = pos_contact2_KS0_2D - (posKS0_KS0_KSGj + posKS0_KSGj_KS_Fj);
    posKSGj_contact2_KS0_KSGj = R_0Gj_contact2(1:2,1:2)' * posKS0_contact2_KS0_KSGj;
    s2 = posKSGj_contact2_KS0_KSGj(1)/param.l_all(2);
    Fext_link2 = frame_contact2 * Fext_link2_KSContactframe;
    Fext_link2(3)=0;       
end

== matlab function PR_Planar_Testbench_2018/DirectDynamics_MuJoCo/KollisionsJacobi1 ==
  data: qj_rad input; dqj_rad input; xEE_ist_3D input; dxEE_3D input; chain_segment input; whichchain input; Jinv_hqx input; Jhred_xqa input; param parameter; n input; location_contact1 input; location_contact2 input; Jac_xpq_contact1 output; Fext_link1 input; Fext_link2 input; Fext_mP_contact1_KS0 output; Tauext_contact1 output; Jac_xpq_contact2 output; Fext_mP_contact2_KS0 output; Tauext_contact2 output; geom2 input size=[4,1]
function [Jac_xpq_contact1, Fext_mP_contact1_KS0, Tauext_contact1, ...
          Jac_xpq_contact2, Fext_mP_contact2_KS0, Tauext_contact2]...
    = fcn(qj_rad, dqj_rad, xEE_ist_3D, dxEE_3D, chain_segment, whichchain, ...
          Jinv_hqx, Jhred_xqa, param, n, location_contact1, location_contact2, Fext_link1, Fext_link2, geom2)
    % Funktion für die Berechnung der Kontaktjacobi-Matrizen, Kontaktkräfte in Plattform- und angetriebenen Gelenkkordinaten
    % Eingabe:
    % qj_rad: Vektor der Gelenkkoordinaten (9x1)
    % dqj_rad: Vektor der Gelenkgeschwindigkeiten (9x1)
    % xEE_ist_3D: Vektor der Plattformkoordinaten (3x1)
    % dxEE_3D: Vektor der Plattformgeschwindigkeiten (3x1)
    % chain_segment: Betroffenes Segment (1x1)
    % whichchain: Betroffene Beinkette (1x1) 
    % Jinv_hqx: Jacobi-Matrix, um dx auf dq projizieren (9x3)
    % Jhred_xqa: Jacobi-Matrix, um dqa auf dx zu projizieren (3x3)
    % n: Anzahl der Kontakte
    % location_contact1: Längennormierter Ort des ersten Kontaktortes im körperfesten KS (1x1)
    % location_contact2: Längennormierter Ort des zweiten Kontaktortes im körperfesten KS (1x1)
    % Fext_link1: Kontaktkräfte am ersten Kontaktort in KS0 (3x1)
    % Fext_link2: Kontaktkräfte am ersten Kontaktort in KS0 (3x1)
    % geom2: Index der zweiten Kontaktgeometrie, die Kraft zeigt von Geometrie 1 zu Geometrie 2 (nx1)
    %
    % Ausgabe:
    % Jac_xpq_contact1: Kontaktjacobi-Matrix, um dq auf dxp am ersten Kontaktort projizieren (3x9)
    % Fext_mP_contact1_KS0: Externe Kräfte und Momente in Plattformkoordinaten und verursacht am ersten Kontaktort (3x1)
    % Tauext_contact1: Externe Momente in Antriebskoordinaten und verursacht am ersten Kontaktort (3x1)
    % Jac_xpq_contact2: Kontaktjacobi-Matrix, um dq auf dxp am ersten Kontaktort projizieren (3x9)
    % Fext_mP_contact2_KS0: Externe Kräfte und Momente in Plattformkoordinaten und verursacht am ersten Kontaktort (3x1)
    % Tauext_contact2: Externe Momente in Antriebskoordinaten und verursacht am ersten Kontaktort (3x1)
    
    % Aran Mohammad, aran.mohammad@imes.uni-hannover.de, 2022-12
    % (C) Institut für Mechatronische Systeme, Universität Hannover

Jac_xpq_contact1 = zeros(3,9);
Fext_mP_contact1_KS0 = zeros(3,1);
Tauext_contact1 = zeros(3,1);
Jac_xpq_contact2 = zeros(3,9);
Fext_mP_contact2_KS0 = zeros(3,1); 
Tauext_contact2 = zeros(3,1);        

if n==1 && ismember( 17, geom2)
    Fext_mP_contact1_KS0 = Fext_link1;
    Tauext_contact1 = Jhred_xqa' * Fext_mP_contact1_KS0;
end

if n == 1 && ~ismember( 17, geom2)
    [~, ~, ~, Jac_xpq_contact1, ~, ~, ~, ~, ~, ~]... 
        = calcJac_colSeg(chain_segment, qj_rad, dqj_rad, xEE_ist_3D, dxEE_3D, param.l_all, param.r_BasisPla_MobPla, ...
                         param.l_all_id, param.r_fixPlat_j, param.r_mobPlat_j, whichchain, location_contact1, 0);
    J_xpx_contact1 = Jac_xpq_contact1 * Jinv_hqx;
    Fext_mP_contact1_KS0 = J_xpx_contact1' * Fext_link1;
    Tauext_contact1 = Jhred_xqa' * Fext_mP_contact1_KS0;
end

if n == 2
    
    [~, ~, ~, Jac_xpq_contact1, ~, ~, ~, ~, ~, ~]... 
        = calcJac_colSeg(1, qj_rad, dqj_rad, xEE_ist_3D, dxEE_3D, param.l_all, param.r_BasisPla_MobPla, ...
                         param.l_all_id, param.r_fixPlat_j, param.r_mobPlat_j, whichchain, location_contact1, 0);
    J_xpx_contact1 = Jac_xpq_contact1 * Jinv_hqx;
    Fext_mP_contact1_KS0 = J_xpx_contact1' * Fext_link1;
    Tauext_contact1 = Jhred_xqa' * Fext_mP_contact1_KS0;
    
   [~, ~, ~, Jac_xpq_contact2, ~, ~, ~, ~, ~, ~]... 
        = calcJac_colSeg(2, qj_rad, dqj_rad, xEE_ist_3D, dxEE_3D, param.l_all, param.r_BasisPla_MobPla, ...
                         param.l_all_id, param.r_fixPlat_j, param.r_mobPlat_j, whichchain, location_contact2, 0);
    J_xpx_contact2 = Jac_xpq_contact2 * Jinv_hqx;
    Fext_mP_contact2_KS0 = J_xpx_contact2' * Fext_link2;
    Tauext_contact2 = Jhred_xqa' * Fext_mP_contact2_KS0;
end

== matlab function PR_Planar_Testbench_2018/Logic/Validation of the EE end target pose/taskspace_limitation ==
  data: xe input; euclid_valid output; ye input; phie input; param parameter
function euclid_valid = fcn(xe,ye, phie, param)
r = sqrt(xe^2+ye^2);

if r <= param.max_radius && abs(phie)< param.max_phie
    euclid_valid = true;
else
    euclid_valid = false;
end

== matlab function PR_Planar_Testbench_2018/DirectDynamics_MuJoCo/MATLAB Function ==
  data: n input; geom1_input input size=[4,1]; n_link output; geom2_input input size=[4,1]; n_chain output
function [n_link, n_chain] = fcn(n, geom1_input, geom2_input)
    % Funktion für die Bestimmung der betroffenen Beinkette und Segmente
    % Eingabe:
    % n: Anzahl der Kontakte
    % geom1_input: Index der ersten Kontaktgeometrie (nx1)
    % geom2_input: Index der zweiten Kontaktgeometrie, die Kraft zeigt von Geometrie 1 zu Geometrie 2 (nx1)
    %
    % Ausgabe:
    % n_link: Betroffenes Segment, 1 oder 2 (1x1)
    % n_chain: Betroffene Beinkette, 1,2,3 (1x1)
    
    % Aran Mohammad, aran.mohammad@imes.uni-hannover.de, 2022-12
    % (C) Institut für Mechatronische Systeme, Universität Hannover

n_link = 0;
n_chain = 0;

geom1 = geom1_input;
geom2 = geom2_input;

% C1L1 = 7   | C1L2 = 11
% C2L1 = 21  | C2L2 = 25
% C3L1 = 31  | C3L2 = 35
% mP = 17
if n == 1
    %C1
    if ismember( 7, geom2)
        n_chain = 1; 
        n_link = 1;
    elseif ismember(11,geom2)
        n_chain = 1;
        n_link = 2;
    
    % C2
    elseif ismember( 21, geom2)
        n_chain = 2; 
        n_link = 1;
    elseif ismember(25,geom2)
        n_chain = 2;
        n_link = 2;
    
    % C3
    elseif ismember( 31, geom2)
        n_chain = 3; 
        n_link = 1;
    elseif ismember(35,geom2)
        n_chain = 3;
        n_link = 2;
    end   
elseif n == 2
    
    if ismember([7,11], geom2)
        n_chain = 1;
    elseif ismember([21,25], geom2)
        n_chain = 2;
    elseif ismember([31,35], geom2)
        n_chain = 3;
    end
end

== matlab function PR_Planar_Testbench_2018/Communication/MATLAB Function1 ==
  data: target input; R_0Gj input; xEE_ist input; FMext_mobPlat_mess_KS0 output; Jxpx_contact1 input; FMext_link_KSSensor input; anre_Achse input
function FMext_mobPlat_mess_KS0 = fcn(target, R_0Gj, xEE_ist, Jxpx_contact1, FMext_link_KSSensor, anre_Achse)

if target ~= 7 % KMS an Link (Achtung: Annahme, dass KMS immer an linker Seite des Links mit Kabel nach unten zeigend montiert ist)
    % KMS immer an linker Seite des Links mit Kabel nach unten zeigend montiert ist
    FMext_KSGj = [FMext_link_KSSensor(1); FMext_link_KSSensor(3); -FMext_link_KSSensor(5)];
    % KMS immer an rechter Seite des Links mit Kabel seitlich nach vorn zeigend montiert ist
%     FMext_KSGj = [FMext_link_KSSensor(1); -FMext_link_KSSensor(3); FMext_link_KSSensor(5)];    
    FMext_link_mess_KS0 = R_0Gj * FMext_KSGj;
    FMext_mobPlat_mess_KS0 = Jxpx_contact1' * FMext_link_mess_KS0; 
else % KMS an mobiler Plattform
    R_0P = [cos(xEE_ist(3)) -sin(xEE_ist(3)) 0;...
            sin(xEE_ist(3))  cos(xEE_ist(3)) 0;...
            0                0               1];
    if anre_Achse == 1
        % KMS an der Seite richtung negativer x-Achse    
        FMext_mobPlat_mess_KS0 = R_0P*[-FMext_link_KSSensor(3); -FMext_link_KSSensor(2); -FMext_link_KSSensor(4)];  
    else
        % KMS an der Seite richtung positiver y-Achse
        FMext_mobPlat_mess_KS0 = R_0P*[-FMext_link_KSSensor(2); FMext_link_KSSensor(3); -FMext_link_KSSensor(4)];
    end
    return
end

== matlab function PR_Planar_Testbench_2018/DirectDynamics_MuJoCo/MATLAB Function2 ==
  data: q_ input; q output; dq_ input; ddq_ input; dq output; ddq output; x output; dx output; ddx output
function [q, dq, ddq, x, dx, ddx] = fcn(q_, dq_, ddq_)
    % Funktion für die Sortierung der Mujoco-Größen
    % Eingabe:
    % q_ in m und rad: Vektor der Gelenk- und Plattformkoordinaten (12x1)
    % qd_ in m/s und rad/s: Vektor der Gelenk- und Plattformgeschwindigkeiten (12x1)
    % qdd_ in m/s^2 und rad/s^2: Vektor der Gelenk- und Plattformbeschleunigungen (12x1)
    %
    % Ausgabe:
    % q in rad: Vektor der Plattformkoordinaten (9x1)
    % dq in rad/s: Vektor der Plattformgeschwindigkeiten (9x1)
    % ddq in rad/s^2: Vektor der Plattformbeschleunigungen (9x1)
    % x in m und rad: Vektor der Plattformkoordinaten (3x1)
    % dx in m/s und rad/s: Vektor der Plattformgeschwindigkeiten (3x1)
    % ddx in m/s^2 und rad/s^2: Vektor der Plattformbeschleunigungen (3x1)
    
    % Aran Mohammad, aran.mohammad@imes.uni-hannover.de, 2022-12
    % (C) Institut für Mechatronische Systeme, Universität Hannover

q = q_([1 2 3 7 8 9 10 11 12]);
x = q_([4 5 6]);

dq = dq_([1 2 3 7 8 9 10 11 12]);
dx = dq_([4 5 6]);

ddq = ddq_([1 2 3 7 8 9 10 11 12]);
ddx = ddq_([4 5 6]);

== matlab function PR_Planar_Testbench_2018/Communication/voltage2force_torque/mittelwert1 ==
  data: u input; y output; set_zero input; mittelwert output
function [y,mittelwert] = mittelwert(u, set_zero)
%#eml
persistent zustand;
persistent mittelwert_z;
persistent i;
if isempty(zustand)
    zustand = 0.0;
    i=1;
    mittelwert_z = 0.0;
end;

if set_zero == 1 && zustand == 0
    zustand = 1;
    mittelwert_z = 0.0;
    i = 1;
elseif set_zero == 0 
    zustand = 0;
end;
    
if zustand == 1
        mittelwert_z = (mittelwert_z * (i-1) + u)/i;
        i=i+1;
end;

y = u - mittelwert_z;
mittelwert = mittelwert_z;

== matlab function PR_Planar_Testbench_2018/Communication/voltage2force_torque/mittelwert2 ==
  data: u input; y output; set_zero input; mittelwert output
function [y,mittelwert] = mittelwert(u, set_zero)
%#eml
persistent zustand;
persistent mittelwert_z;
persistent i;
if isempty(zustand)
    zustand = 0.0;
    i=1;
    mittelwert_z = 0.0;
end;

if set_zero == 1 && zustand == 0
    zustand = 1;
    mittelwert_z = 0.0;
    i = 1;
elseif set_zero == 0 
    zustand = 0;
end;
    
if zustand == 1
        mittelwert_z = (mittelwert_z * (i-1) + u)/i;
        i=i+1;
end;

y = u - mittelwert_z;
mittelwert = mittelwert_z;

== matlab function PR_Planar_Testbench_2018/Communication/voltage2force_torque/mittelwert3 ==
  data: u input; y output; set_zero input; mittelwert output
function [y,mittelwert] = mittelwert(u, set_zero)
%#eml
persistent zustand;
persistent mittelwert_z;
persistent i;
if isempty(zustand)
    zustand = 0.0;
    i=1;
    mittelwert_z = 0.0;
end;

if set_zero == 1 && zustand == 0
    zustand = 1;
    mittelwert_z = 0.0;
    i = 1;
elseif set_zero == 0 
    zustand = 0;
end;
    
if zustand == 1
        mittelwert_z = (mittelwert_z * (i-1) + u)/i;
        i=i+1;
end;

y = u - mittelwert_z;
mittelwert = mittelwert_z;

== matlab function PR_Planar_Testbench_2018/Communication/voltage2force_torque/mittelwert4 ==
  data: u input; y output; set_zero input; mittelwert output
function [y,mittelwert] = mittelwert(u, set_zero)
%#eml
persistent zustand;
persistent mittelwert_z;
persistent i;
if isempty(zustand)
    zustand = 0.0;
    i=1;
    mittelwert_z = 0.0;
end;

if set_zero == 1 && zustand == 0
    zustand = 1;
    mittelwert_z = 0.0;
    i = 1;
elseif set_zero == 0 
    zustand = 0;
end;
    
if zustand == 1
        mittelwert_z = (mittelwert_z * (i-1) + u)/i;
        i=i+1;
end;

y = u - mittelwert_z;
mittelwert = mittelwert_z;

== matlab function PR_Planar_Testbench_2018/Communication/voltage2force_torque/mittelwert5 ==
  data: u input; y output; set_zero input; mittelwert output
function [y,mittelwert] = mittelwert(u, set_zero)
%#codegen
persistent zustand;
persistent mittelwert_z;
persistent i;
if isempty(zustand)
    zustand = 0.0;
    i=1;
    mittelwert_z = 0.0;
end;

if set_zero == 1 && zustand == 0
    zustand = 1;
    mittelwert_z = 0.0;
    i = 1;
elseif set_zero == 0 
    zustand = 0;
end;
    
if zustand == 1
        mittelwert_z = (mittelwert_z * (i-1) + u)/i;
        i=i+1;
end;

y = u - mittelwert_z;
mittelwert = mittelwert_z;

== matlab function PR_Planar_Testbench_2018/Communication/voltage2force_torque/mittelwet2 ==
  data: u input; y output; set_zero input; mittelwert output
function [y,mittelwert] = mittelwert(u, set_zero)
%#eml
persistent zustand;
persistent mittelwert_z;
persistent i;
if isempty(zustand)
    zustand = 0.0;
    i=1;
    mittelwert_z = 0.0;
end;

if set_zero == 1 && zustand == 0
    zustand = 1;
    mittelwert_z = 0.0;
    i = 1;
elseif set_zero == 0 
    zustand = 0;
end;
    
if zustand == 1
        mittelwert_z = (mittelwert_z * (i-1) + u)/i;
        i=i+1;
end;

y = u - mittelwert_z;
mittelwert = mittelwert_z;
